simulink model "Inverse_geometry"  (R2025b)
settings: Solver=VariableStepAuto  StartTime=0.0  StopTime=10.0  RelTol=1e-3
model workspace (MAT data in the model file):
  Sig = Simulink.Signal
  Sig.Dimensions = -1
  Sig.DimensionsMode = 'auto'
  Sig.Complexity = 'auto'
  Sig.SampleTime = -1
  Sig.SamplingMode = 'auto'
  Sig.DataType = 'auto'
  beta_array = [-30.0099338385 -28.4709894525 -26.9233449828 -25.3669017656 -23.8015796232 -22.2273180918 -20.6440777542 -19.0518416802 -17.450616983 -15.8404364944 -14.2213605679 -12.5934790137 -10.9569131737 -9.31181814393 -7.65838515061 -5.99684408827 -4.32746622757 -2.65056710008 -0.966509567874 0.724292915289 2.42137284465 4.12420500193 5.83220258594 7.5447131351 9.26101424368 10.9803090779 12.7017217034 14.4242922434 16.1469718952 17.8686178448 19.5879881357 21.3037365625 23.0144076867 24.7184320944 26.4141220517 28.0996677462 29.7731343488 31.4324601733 33.075456263 34.6998077837]
  x_actuator = [-20 -18.9230769231 -17.8461538462 -16.7692307692 -15.6923076923 -14.6153846154 -13.5384615385 -12.4615384615 -11.3846153846 -10.3076923077 -9.23076923077 -8.15384615385 -7.07692307692 -6 -4.92307692308 -3.84615384615 -2.76923076923 -1.69230769231 -0.615384615385 0.461538461538 1.53846153846 2.61538461538 3.69230769231 4.76923076923 5.84615384615 6.92307692308 8 9.07692307692 10.1538461538 11.2307692308 12.3076923077 13.3846153846 14.4615384615 15.5384615385 16.6153846154 17.6923076923 18.7692307692 19.8461538462 20.9230769231 22]
settings Model: Creator=mikol  LastModifiedBy=ikita

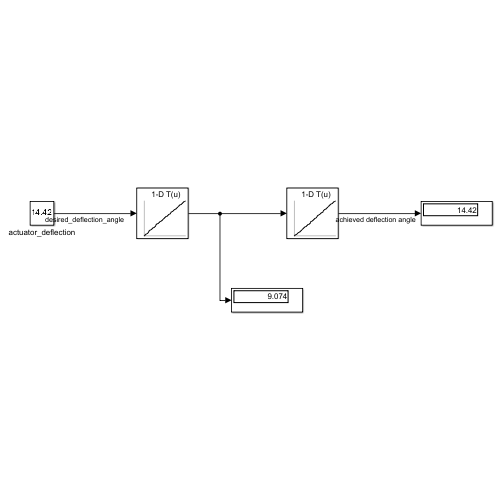
[thumbnail: Simulink's stored preview of the top-level diagram]
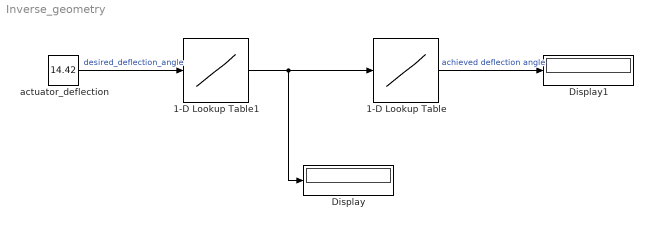
== system Inverse_geometry ==
  1-D Lookup Table : Lookup_n-D  NumberOfTableDimensions=1  BreakpointsForDimension1=x_actuator  Table=beta_array  InternalRulePriority=Speed  RndMeth=Simplest
  1-D Lookup Table1 : Lookup_n-D  NumberOfTableDimensions=1  BreakpointsForDimension1=beta_array  Table=x_actuator  InternalRulePriority=Speed  RndMeth=Simplest
  Display : Display
  Display1 : Display
  actuator_deflection : Constant  Value=14.42
  wires:
  1-D Lookup Table1/1 -> Display/1, 1-D Lookup Table/1
  actuator_deflection/1 -> 1-D Lookup Table1/1  "desired_deflection_angle"
  1-D Lookup Table/1 -> Display1/1  "achieved deflection angle"
